simulink model "TestForce"  (R2022b)
settings: Solver=FixedStepAuto  StartTime=0.0  StopTime=5  FixedStep=simulator.TimeStep  RelTol=1e-3  EnableMultiTasking=on
settings Model: Creator=At  LastModifiedBy=ateay
settings SolverCC: ConcurrentTasks=on  AlgebraicLoopSolver=TrustRegion  InsertRTBMode=Never (minimum delay)
settings DataIOCC: SaveFormat=StructureWithTime  ReturnWorkspaceOutputs=off
settings OptimizationCC: BlockReduction=off  OptimizeBlockIOStorage=off  BufferReuse=off  GlobalBufferReuse=off  ExpressionFolding=off  LocalBlockOutputs=off
settings DebuggingCC: UnconnectedInputMsg=warning  UnconnectedOutputMsg=warning  UnconnectedLineMsg=warning  SFMachineParentedDataDiag=warning  ArithmeticOperatorsInVariantConditions=warning
settings HardwareCC: ProdBitPerPointer=32  ProdBitPerSizeT=32  ProdBitPerPtrDiffT=32  ProdLargestAtomicFloat=None  ProdWordSize=32  ProdLongLongMode=on  ProdHWDeviceType=Generic->32-bit x86 compatible
settings ModelReferenceCC: EnableRefExpFcnMdlSchedulingChecks=on  ModelReferenceNumInstancesAllowed=Single
settings SFSimCC: SimUseLocalCustomCode=off  CustomCodeUndefinedFunction=UseInterfaceOnly
settings RTWCC: Description=Simulink Real-Time  SystemTargetFile=slrt.tlc  TemplateMakefile=slrt_default_tmf  RTWUseLocalCustomCode=off  RTWCompilerOptimization=on
settings CodeAppCC: StateflowObjectComments=on
settings SimulinkRealTimeCC: OptimizeReductions=off  RL32LogBufSizeModifier=1000000

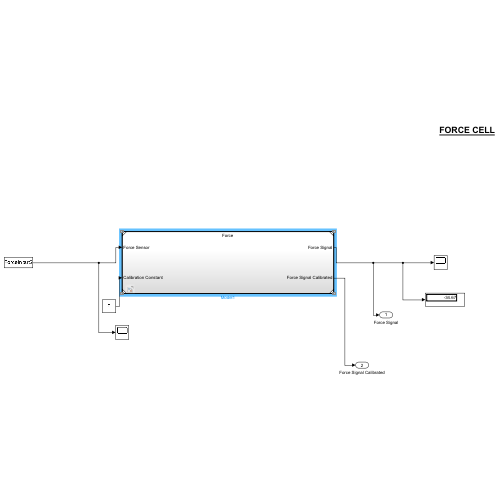
[thumbnail: Simulink's stored preview of the top-level diagram]
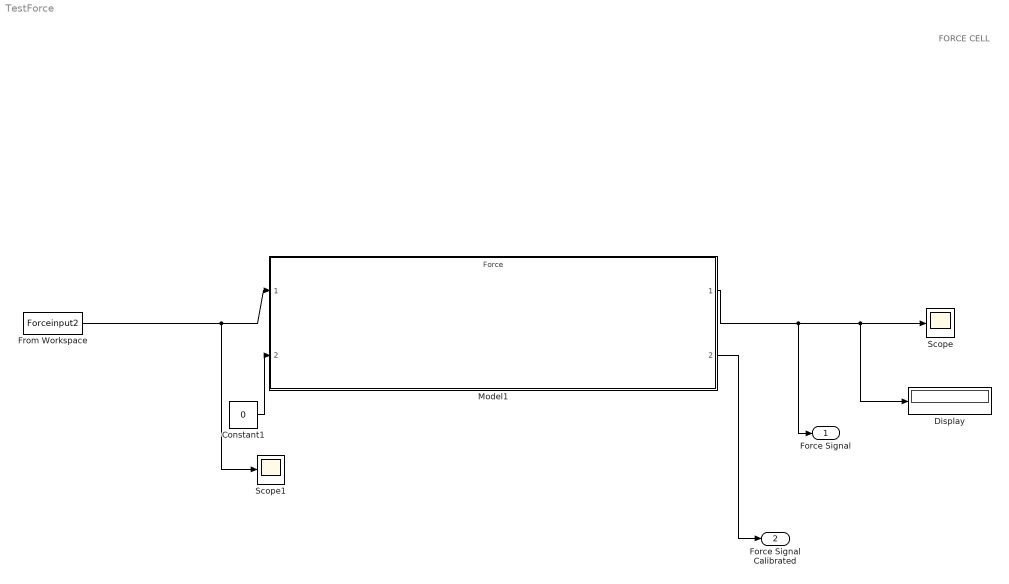
== system TestForce ==
  note: FORCE CELL
  Constant1 : Constant  Value=0
  Display : Display
  From Workspace : FromWorkspace  VariableName=Forceinput2
  Model1 : ModelReference  ModelNameDialog=Force.slx  SimulationMode=Normal  ModelReferenceVersion=1.61
  Scope : Scope
  Scope1 : Scope
  Force Signal : Outport
  Force Signal Calibrated : Outport  Port=2
  wires:
  Model1/1 -> Force Signal/1, Display/1, Scope/1
  From Workspace/1 -> Scope1/1, Model1/1
  Constant1/1 -> Model1/2
  Model1/2 -> Force Signal Calibrated/1
